simulink model "Lab06B"  (R2021a)
settings: Solver=VariableStepAuto  StartTime=0.0  StopTime=10.0  RelTol=1e-3  EnableMultiTasking=on
settings Model: Creator=Student  LastModifiedBy=shirs
settings SolverCC: AlgebraicLoopSolver=TrustRegion
settings DataIOCC: ReturnWorkspaceOutputs=off
settings OptimizationCC: LifeSpan=inf
settings DebuggingCC: SFUnexpectedBacktrackingDiag=warning  SFNoUnconditionalDefaultTransitionDiag=warning  SFMachineParentedDataDiag=warning  ArithmeticOperatorsInVariantConditions=warning
settings SFSimCC: SimUseLocalCustomCode=off  CustomCodeUndefinedFunction=UseInterfaceOnly
settings RTWCC: RTWUseLocalCustomCode=off
settings CodeAppCC: StateflowObjectComments=on
settings GRTTargetCC: TargetLangStandard=C89/C90 (ANSI)
settings ConfigComp: CovMetricSettings=dw  CovSaveCumulativeToWorkspaceVar=on  CovSaveSingleToWorkspaceVar=on  CovExternalEMLEnable=off

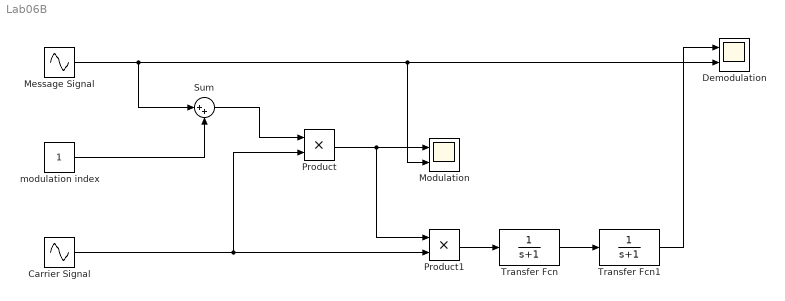
== system Lab06B ==
  Carrier Signal : Sin  Frequency=157.08  SampleTime=0.0002
  Demodulation : Scope  NumInputPorts=2
  Message Signal : Sin  Frequency=6.28  SampleTime=0.0002
  Modulation : Scope  NumInputPorts=2
  Product : Product
  Product1 : Product
  Sum : Sum  Inputs=|++
  Transfer Fcn : TransferFcn  Denominator=[1 1]
  Transfer Fcn1 : TransferFcn  Denominator=[1 1]
  modulation index : Constant
  wires:
  modulation index/1 -> Sum/2
  Sum/1 -> Product/1
  Carrier Signal/1 -> Product1/2, Product/2
  Product1/1 -> Transfer Fcn/1
  Transfer Fcn/1 -> Transfer Fcn1/1
  Transfer Fcn1/1 -> Demodulation/1
  Message Signal/1 -> Sum/1, Modulation/2, Demodulation/2
  Product/1 -> Product1/1, Modulation/1
